simulink model "servoPDF"  (R2023b)
settings: Solver=ode1  StartTime=0.0  StopTime=t_run+2  FixedStep=0.001  RelTol=1e-3  EnableMultiTasking=on
PostLoadFcn:
  | kp = 4; kd = 0.2
  | pf = 200;
  | 
  | t_run = 5;
InitFcn:
  | %PDdesign
undefined symbols (not defined in the file or in its folder): HIL
libraries: quarc_library x5, simulink x2
settings Model: ExtModeTrigDuration=20000  Creator=jpineros  LastModifiedBy=labuser
settings SolverCC: AlgebraicLoopSolver=TrustRegion  PositivePriorityOrder=on  AutoInsertRateTranBlk=on
settings DataIOCC: SaveOutput=off  SignalLogging=off  DSMLogging=off  SaveTime=off  ReturnWorkspaceOutputs=off
settings DebuggingCC: UnconnectedInputMsg=warning  UnconnectedOutputMsg=warning  UnconnectedLineMsg=warning  ArithmeticOperatorsInVariantConditions=warning
settings HardwareCC: ProdBitPerPointer=32  ProdBitPerSizeT=32  ProdBitPerPtrDiffT=32  ProdLargestAtomicInteger=Long  ProdWordSize=32  ProdHWDeviceType=ARM Compatible->ARM 7
settings ModelReferenceCC: EnableRefExpFcnMdlSchedulingChecks=on
settings SFSimCC: SimUseLocalCustomCode=off  CustomCodeUndefinedFunction=UseInterfaceOnly
settings RTWCC: Description=QUARC Linux RT ARMv7 Target (NI ELVIS III, NI myRIO) Using Toolchain  SystemTargetFile=quarc_linux_rt_armv7.tlc  TemplateMakefile=quarc_default_tmf  RTWUseLocalCustomCode=off  Toolchain=QUARC linux_rt_armv7 | gmake (64-bit Windows)  BuildConfiguration=Faster Runs
settings CodeAppCC: StateflowObjectComments=on
settings STFCustomTargetCC: ConcurrentExecutionCompliant=on  MatFileLogging=on  GRTInterface=on  UseToolchainInfoCompliant=on  SystemTargetFile=quarc_linux_rt_armv7.tlc
settings GRTTargetCC: ParMdlRefBuildCompliant=off  CompOptLevelCompliant=off  CombineOutputUpdateFcns=off  CPPClassGenCompliant=off  GRTInterface=on  ExtMode=on  ExtModeMexFile=quarc_comm  ExtModeMexArgs='-t tcpip://172.22.11.10:17000?keep_alive=1 ','tcpip://172.22.11.10:17000'

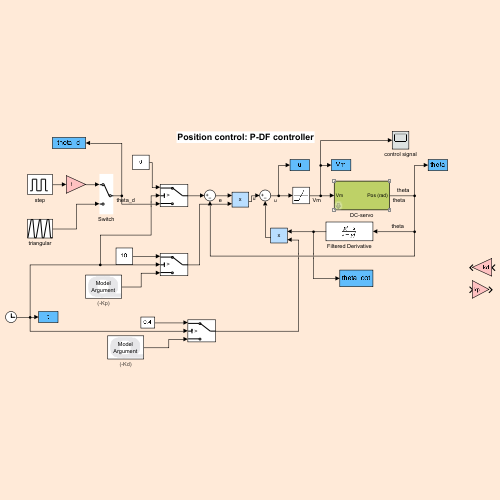
[thumbnail: Simulink's stored preview of the top-level diagram]
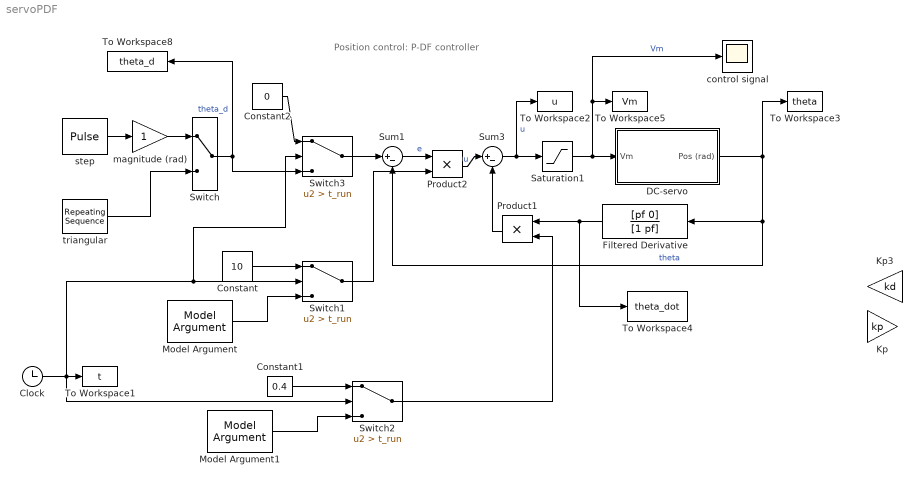
== system servoPDF ==
  note: Position control: P-DF controller
  Clock : Clock
  Constant : Constant  Value=10
  Constant1 : Constant  Value=0.4
  Constant2 : Constant  Value=0
  DC-servo : Subsystem
  Filtered Derivative : TransferFcn  Numerator=[pf 0]  Denominator=[1 pf]
  Kp : Gain  Gain=kp
  Kp3 : Gain  Gain=kd
  Model Argument : quarc_library/Sources/Signals/Model Argument  argument_name=Kp  has_value=on  data_type_mode=Specify via dialog  data_type=double  max_length=80  default_value=kp  variable_size=on
      settings: AttributesFormatString=(-%<argument_name>)  SourceProductName=QUARC Targets
  Model Argument1 : quarc_library/Sources/Signals/Model Argument  argument_name=Kd  has_value=on  data_type_mode=Specify via dialog  data_type=double  max_length=80  default_value=kd  variable_size=on
      settings: AttributesFormatString=(-%<argument_name>)  SourceProductName=QUARC Targets
  Product1 : Product
  Product2 : Product
  Saturation1 : Saturate  UpperLimit=5  LowerLimit=-5
  Sum1 : Sum  Inputs=|+-
  Sum3 : Sum  Inputs=|+-
  Switch : ManualSwitch
  Switch1 : Switch  Criteria=u2 > Threshold  Threshold=t_run  SaturateOnIntegerOverflow=off  InputSameDT=off
  Switch2 : Switch  Criteria=u2 > Threshold  Threshold=t_run  SaturateOnIntegerOverflow=off  InputSameDT=off
  Switch3 : Switch  Criteria=u2 > Threshold  Threshold=t_run  SaturateOnIntegerOverflow=off  InputSameDT=off
  To Workspace1 : ToWorkspace  VariableName=t  SampleTime=-1
  To Workspace2 : ToWorkspace  VariableName=u  SampleTime=-1
  To Workspace3 : ToWorkspace  VariableName=theta  SampleTime=-1
  To Workspace4 : ToWorkspace  VariableName=theta_dot  SampleTime=-1
  To Workspace5 : ToWorkspace  VariableName=Vm  SampleTime=-1
  To Workspace8 : ToWorkspace  VariableName=theta_d  SampleTime=-1
  control signal : Scope
  magnitude (rad) : Gain
  step : DiscretePulseGenerator  PulseType=Time based  PulseWidth=50
  triangular : simulink/Sources/Repeating Sequence  rep_seq_t=[0 0.4 0.6 0.8 1]  rep_seq_y="[0 1 1  0 0]*6"
  wires:
  Clock/1 -> Switch2/2, Switch3/2, Switch1/2, To Workspace1/1
  step/1 -> magnitude (rad)/1
  DC-servo/1(Pos (rad)) -> To Workspace3/1, Filtered Derivative/1, Sum1/2  "theta"
  Sum1/1 -> Product2/1  "e"
  Saturation1/1 -> control signal/1, To Workspace5/1, DC-servo/1(Vm)  "Vm"
  Switch/1 -> To Workspace8/1, Switch3/3  "theta_d"
  Product1/1 -> Sum3/2
  Filtered Derivative/1 -> To Workspace4/1, Product1/1
  Product2/1 -> Sum3/1  "u"
  Sum3/1 -> To Workspace2/1, Saturation1/1  "u"
  triangular/1 -> Switch/2
  magnitude (rad)/1 -> Switch/1
  Constant/1 -> Switch1/1
  Switch1/1 -> Product2/2
  Model Argument/1 -> Switch1/3
  Model Argument1/1 -> Switch2/3
  Switch2/1 -> Product1/2
  Constant1/1 -> Switch2/1
  Switch3/1 -> Sum1/1
  Constant2/1 -> Switch3/1

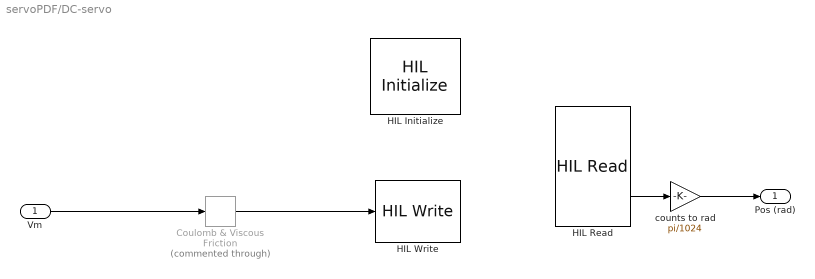
== system servoPDF/DC-servo ==
  Vm : Inport
  Coulomb & Viscous Friction : simulink/Discontinuities/Coulomb & Viscous Friction  Commented=through  offset=[0.08]  gain=1
  HIL Initialize : quarc_library/Data Acquisition/Generic/Configuration/HIL Initialize  object_name=HIL-1  board_type=qab_controls  board_number=0  board_options=""  exclusive=off  active=on  hardware_clocks=[]  clock_modes=[]  initial_clock_frequencies=[]  set_clock_params_at_start=off  set_clock_params_at_switch_in=off  set_clock_frequencies_at_start=off  set_clock_frequencies_at_switch_in=off  analog_input_channels=[0]  analog_input_configurations=[]  analog_input_maximums=[10]  analog_input_minimums=[-10]  set_analog_input_params_at_start=off  set_analog_input_params_at_switch_in=off  analog_output_channels=[0]  analog_output_maximums=[5]  analog_output_minimums=[-5]  initial_analog_outputs=[0]  final_analog_outputs=[0]  watchdog_analog_outputs=[]  set_analog_output_params_at_start=off  set_analog_output_params_at_switch_in=off  set_analog_outputs_at_start=on  set_analog_outputs_at_switch_in=off  set_analog_outputs_at_terminate=on  set_analog_outputs_at_switch_out=off  set_analog_outputs_on_watchdog=off  digital_input_channels=[]  digital_output_channels=[0]  digital_output_configuration=[]  initial_digital_outputs=[1]  final_digital_outputs=[0]  watchdog_digital_outputs=[]  set_digital_output_params_at_start=off  set_digital_output_params_at_switch_in=off  set_digital_outputs_at_start=on  set_digital_outputs_at_switch_in=off  set_digital_outputs_at_terminate=on  set_digital_outputs_at_switch_out=off  set_digital_outputs_on_watchdog=off  encoder_channels=[0:1]  quadrature=[4]  encoder_filter_frequency=[]  initial_encoder_counts=[0]  set_encoder_params_at_start=off  set_encoder_params_at_switch_in=off  set_encoder_counts_at_start=on  set_encoder_counts_at_switch_in=off  pwm_channels=[0]  pwm_modes=0  pwm_frequency=40e6/2047  pwm_configuration=[1]  pwm_alignment=[0]  pwm_polarity=[1]  pwm_leading_deadband=[0]  pwm_trailing_deadband=[0]  initial_pwm_outputs=[0]  final_pwm_outputs=[0]  watchdog_pwm_outputs=[]  set_pwm_params_at_start=off  set_pwm_params_at_switch_in=off  set_pwm_outputs_at_start=on  set_pwm_outputs_at_switch_in=off  set_pwm_outputs_at_terminate=on  set_pwm_outputs_at_switch_out=off  set_pwm_outputs_on_watchdog=off  other_output_channels=[]  initial_other_outputs=[]  final_other_outputs=[]  watchdog_other_outputs=[]  set_other_outputs_at_start=off  set_other_outputs_at_switch_in=off  set_other_outputs_at_terminate=off  set_other_outputs_at_switch_out=off  set_other_outputs_on_watchdog=off
  HIL Read : quarc_library/Data Acquisition/Generic/Immediate I//O/HIL Read  object_name=HIL-1  analog_channels=0  encoder_channels=[0]  digital_channels=[]  other_channels=[]  sample_time=qc_get_step_size  active=on  vector_output=off  data_type_mode=Inherit via back propagation  encoder_data_type=double  digital_data_type=boolean
  HIL Write : quarc_library/Data Acquisition/Generic/Immediate I//O/HIL Write  object_name=HIL-1  analog_channels=0  pwm_channels=[]  digital_channels=[]  other_channels=[]  sample_time=-1  active=off  vector_input=off
  counts to rad : Gain  Gain=pi/1024
  Pos (rad) : Outport
  wires:
  HIL Read/2 -> counts to rad/1
  Vm/1 -> Coulomb & Viscous Friction/1
  counts to rad/1 -> Pos (rad)/1
  Coulomb & Viscous Friction/1 -> HIL Write/1
